simulink model "spring_mass_model_01"  (R2014a)
settings: Solver=FixedStepDiscrete  StartTime=0.0  StopTime=inf  FixedStep=sample_time  RelTol=1e-3
values from neighbouring files (symbols this model uses):
  sample_time = 1/update_freq    (= 0.001)    [init_spring_mass_model_01.m]
undefined symbols (not defined in the file or in its folder): boom_mount_angle, c_energy, contact_threshold, control_start_time, d_y_boom_com_offset, d_y_boom_hip_offset, d_y_mount_to_com, desired_torso_angle, DiscIntNeverNeededParam, dt_thrust, dx_avg_desired, extra_leg_damping, F_thrust, fcut_contact, ff_energy_l, ff_energy_r, g, g_reduced, h_boom, i_limit_lateral, initial_com_height, initial_dt, initial_dx, j_leg, k0_virtual, k_placement, k_sea, kd_flight, kd_lateral, kd_leg_angle, kd_leg_length_secondary, kd_torso, kd_virtual, ki_lateral, kp_flight_max, kp_flight_min, kp_lateral, kp_leg_angle, kp_leg_length_secondary, kp_torso, kp_virtual, l0_virtual, l_boom, l_boom_projected, l_max, l_min, l_retract, l_seg, lambda1, lambda2, lateral_offset, LEG_MTR_MAX_TORQUE, loaded_threshold, m_leg_motor, m_total_real, max_k_virtual, max_leg_angle, max_torque_lateral, min_k_virtual, min_leg_angle ... (+6)
libraries: simulink x22
(part 2 of 2)

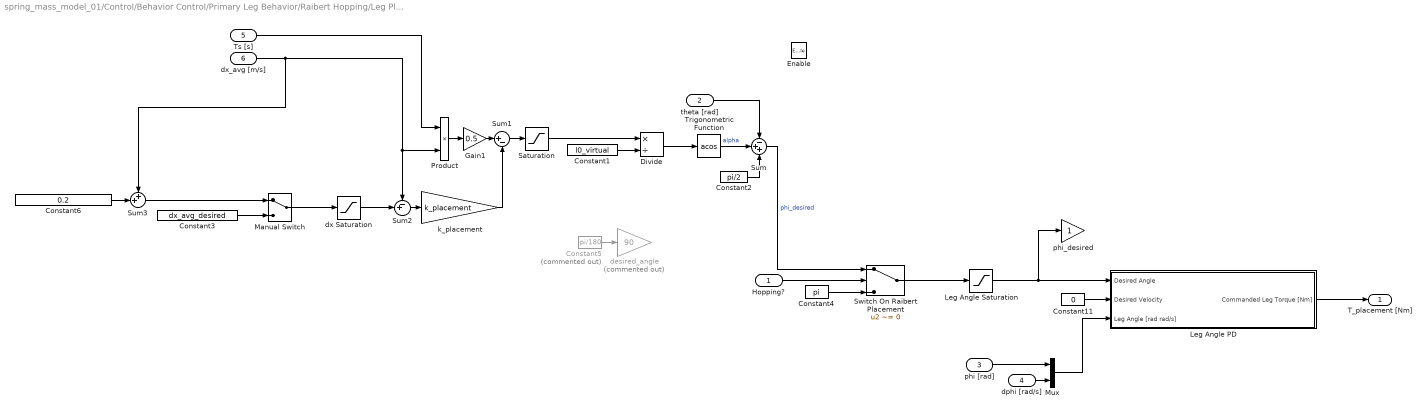
== system spring_mass_model_01/Control/Behavior Control/Primary Leg Behavior/Raibert Hopping/Leg Placement Torque ==
  Hopping? : Inport
  theta [rad] : Inport  Port=2
  phi [rad] : Inport  Port=3
  dphi [rad/s] : Inport  Port=4
  Ts [s] : Inport  Port=5
  dx_avg [m/s] : Inport  Port=6
  Enable : EnablePort  StatesWhenEnabling=reset
  Constant1 : Constant  Value=l0_virtual
  Constant11 : Constant  Value=0
  Constant2 : Constant  Value=pi/2
  Constant3 : Constant  Value=dx_avg_desired
  Constant4 : Constant  Value=pi
  Constant5 : Constant  Commented=on  Value=pi/180
  Constant6 : Constant  Value=0.2
  Divide : Product  Inputs=*/
  Gain1 : Gain  Gain=0.5
  Leg Angle PD : Subsystem
  Leg Angle Saturation : Saturate  UpperLimit=max_leg_angle  LowerLimit=min_leg_angle
      settings: AttributesFormatString=Hi: %<UpperLimit>\nLo: %<LowerLimit>
  Manual Switch : ManualSwitch
  Mux : Mux  Inputs=2
  Product : Product
  Saturation : Saturate  UpperLimit=x_limit  LowerLimit=-x_limit
      settings: AttributesFormatString=Hi: %<UpperLimit>\nLo: %<LowerLimit>
  Sum : Sum  Inputs=-++
  Sum1 : Sum  Inputs=|+-
  Sum2 : Sum  Inputs=-+|
  Sum3 : Sum  Inputs=++|
  Switch On Raibert Placement : Switch  Criteria=u2 ~= 0
  Trigonometric Function : Trigonometry  Operator=acos
  desired_angle : Gain  Commented=on  Gain=90
  dx Saturation : Saturate  UpperLimit=dx_avg_desired  LowerLimit=0
      settings: AttributesFormatString=Hi: %<UpperLimit>\nLo: %<LowerLimit>
  k_placement : Gain  Gain=k_placement
  phi_desired : Gain
  T_placement [Nm] : Outport  OutputWhenDisabled=reset  InitialOutput=[0]
  wires:
  Sum3/1 -> Manual Switch/1
  Constant6/1 -> Sum3/2
  dx_avg [m/s]/1 -> Product/2, Sum2/1, Sum3/1
  Constant3/1 -> Manual Switch/2
  Manual Switch/1 -> dx Saturation/1
  Switch On Raibert Placement/1 -> Leg Angle Saturation/1
  Constant5/1 -> desired_angle/1
  Leg Angle Saturation/1 -> Leg Angle PD/1(Desired Angle), phi_desired/1
  Hopping?/1 -> Switch On Raibert Placement/2
  Constant4/1 -> Switch On Raibert Placement/3
  dx Saturation/1 -> Sum2/2
  Sum2/1 -> k_placement/1
  k_placement/1 -> Sum1/2
  Sum1/1 -> Saturation/1
  Sum/1 -> Switch On Raibert Placement/1  "phi_desired"
  theta [rad]/1 -> Sum/1
  Constant2/1 -> Sum/3
  Trigonometric Function/1 -> Sum/2  "alpha"
  Divide/1 -> Trigonometric Function/1
  Constant1/1 -> Divide/2
  Saturation/1 -> Divide/1
  Gain1/1 -> Sum1/1
  Product/1 -> Gain1/1
  Ts [s]/1 -> Product/1
  dphi [rad/s]/1 -> Mux/2
  phi [rad]/1 -> Mux/1
  Leg Angle PD/1(Commanded Leg Torque [Nm]) -> T_placement [Nm]/1
  Mux/1 -> Leg Angle PD/3(Leg Angle [rad rad/s])
  Constant11/1 -> Leg Angle PD/2(Desired Velocity)

== system spring_mass_model_01/Control/Behavior Control/Primary Leg Behavior/Raibert Hopping/Leg Thrust ==
  Enable : EnablePort  StatesWhenEnabling=reset  ShowOutputPort=on
  F_thrust : Gain  Gain=F_thrust
  Thrust Timer : Subsystem
  thrust period? : simulink/Logic and Bit Operations/Compare To Constant  relop=<=  const=dt_thrust  OutDataTypeStr=uint8
  Thrust [N] : Outport  OutputWhenDisabled=reset  InitialOutput=[0]
  wires:
  thrust period?/1 -> F_thrust/1
  Enable/1 -> Thrust Timer/Enable
  Thrust Timer/1(timer [s]) -> thrust period?/1
  F_thrust/1 -> Thrust [N]/1

== system spring_mass_model_01/Control/Behavior Control/Primary Leg Behavior/Raibert Hopping/Nonlinear Spring Stiffness ==
  Right/Left [1/0] : Inport
  dl_virtual [m/s] : Inport  Port=2
  E_target1 : Constant  Value=ff_energy_r
  E_target2 : Constant  Value=ff_energy_l
  Product : Product  Inputs=3
  Saturation : Saturate  UpperLimit=max_k_virtual  LowerLimit=min_k_virtual  ZeroCross=off
  Sum : Sum  Inputs=+|-
  Sum2 : Sum  Inputs=--|
  Switch1 : Switch  Criteria=u2 ~= 0
  c_energy : Constant  Value=c_energy
  c_energy1 : Constant  Value=raibert_energy_injection
  k0_virtual : Constant  Value=k0_virtual
  k_virtual [N/m] : Outport
  wires:
  Product/1 -> Sum/2
  Sum/1 -> Saturation/1
  Saturation/1 -> k_virtual [N/m]/1
  k0_virtual/1 -> Sum/1
  c_energy/1 -> Product/3
  dl_virtual [m/s]/1 -> Product/2
  E_target1/1 -> Switch1/1
  E_target2/1 -> Switch1/3
  Right/Left [1/0]/1 -> Switch1/2
  Switch1/1 -> Sum2/2
  c_energy1/1 -> Sum2/1
  Sum2/1 -> Product/1

== system spring_mass_model_01/Control/Behavior Control/Primary Leg Behavior/Raibert Hopping/Trunk Balance PD Compensation ==
  Torso Pitch [rad rad/s] : Inport
  Enable : EnablePort  StatesWhenEnabling=reset
  Constant2 : Constant  Value=0
  Demux : Demux  Outputs=2
  Derivative Gain : Gain  Gain=kd_torso
  Gain1 : Gain  Gain=-1
  Proportional Gain : Gain  Gain=kp_torso
  Reference Lean [rad] : Constant  Value=desired_torso_angle
  Sum1 : Sum  Inputs=|+-
  Sum4 : Sum  Inputs=|+-
  Sum5 : Sum
  Torque [Nm] : Outport  OutputWhenDisabled=reset  InitialOutput=[0]
  wires:
  Gain1/1 -> Torque [Nm]/1
  Sum1/1 -> Derivative Gain/1
  Proportional Gain/1 -> Sum5/1
  Derivative Gain/1 -> Sum5/2
  Torso Pitch [rad rad/s]/1 -> Demux/1
  Sum4/1 -> Proportional Gain/1
  Demux/1 -> Sum4/2
  Reference Lean [rad]/1 -> Sum4/1
  Constant2/1 -> Sum1/1
  Demux/2 -> Sum1/2
  Sum5/1 -> Gain1/1

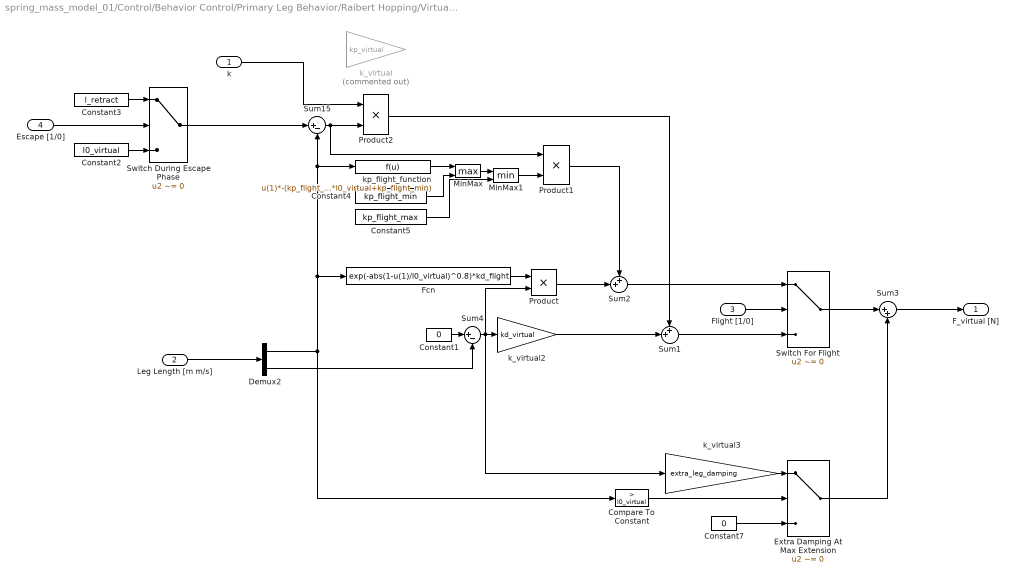
== system spring_mass_model_01/Control/Behavior Control/Primary Leg Behavior/Raibert Hopping/Virtual Leg Force and Swing Leg Retraction ==
  k : Inport
  Leg Length [m m/s] : Inport  Port=2
  Flight [1/0] : Inport  Port=3
  Escape [1/0] : Inport  Port=4
  Compare To Constant : simulink/Logic and Bit Operations/Compare To Constant  relop=>  const=l0_virtual  OutDataTypeStr=boolean
  Constant1 : Constant  Value=0
  Constant2 : Constant  Value=l0_virtual
  Constant3 : Constant  Value=l_retract
  Constant4 : Constant  Value=kp_flight_min
  Constant5 : Constant  Value=kp_flight_max
  Constant7 : Constant  Value=0
  Demux2 : Demux  Outputs=2
  Extra Damping At Max Extension : Switch  Criteria=u2 ~= 0
  Fcn : Fcn  Expr=exp(-abs(1-u(1)/l0_virtual)^0.8)*kd_flight
  MinMax : MinMax  Function=max  Inputs=2
  MinMax1 : MinMax  Inputs=2
  Product : Product
  Product1 : Product
  Product2 : Product
  Sum1 : Sum  Inputs=++|
  Sum15 : Sum  Inputs=|+-
  Sum2 : Sum  Inputs=++|
  Sum3 : Sum  Inputs=|++
  Sum4 : Sum  Inputs=|+-
  Switch During Escape Phase : Switch  Criteria=u2 ~= 0
  Switch For Flight : Switch  Criteria=u2 ~= 0
  k_virtual : Gain  Commented=on  Gain=kp_virtual
  k_virtual2 : Gain  Gain=kd_virtual
  k_virtual3 : Gain  Gain=extra_leg_damping
  kp_flight_function : Fcn  Expr=u(1)*-(kp_flight_max - kp_flight_min)/(l0_virtual - l_min)+((kp_flight_max - kp_flight_min)/(l0_virtual - l_min)*l0_virtual+kp_flight_min)
  F_virtual [N] : Outport
  wires:
  k_virtual3/1 -> Extra Damping At Max Extension/1
  Sum3/1 -> F_virtual [N]/1
  Extra Damping At Max Extension/1 -> Sum3/2
  Constant7/1 -> Extra Damping At Max Extension/3
  Compare To Constant/1 -> Extra Damping At Max Extension/2
  Switch During Escape Phase/1 -> Sum15/1
  Constant5/1 -> MinMax1/2
  MinMax1/1 -> Product1/2
  Constant4/1 -> MinMax/2
  MinMax/1 -> MinMax1/1
  Product1/1 -> Sum2/1
  kp_flight_function/1 -> MinMax/1
  Fcn/1 -> Product/1
  Sum15/1 -> Product2/2, Product1/1
  Leg Length [m m/s]/1 -> Demux2/1
  Demux2/1 -> Compare To Constant/1, Fcn/1, Sum15/2, kp_flight_function/1
  Sum1/1 -> Switch For Flight/3
  Constant1/1 -> Sum4/1
  Demux2/2 -> Sum4/2
  Product2/1 -> Sum1/1
  Sum4/1 -> k_virtual2/1, Product/2, k_virtual3/1
  k_virtual2/1 -> Sum1/2
  Flight [1/0]/1 -> Switch For Flight/2
  Escape [1/0]/1 -> Switch During Escape Phase/2
  Constant2/1 -> Switch During Escape Phase/3
  Constant3/1 -> Switch During Escape Phase/1
  Product/1 -> Sum2/2
  Switch For Flight/1 -> Sum3/1
  Sum2/1 -> Switch For Flight/1
  k/1 -> Product2/1

== system spring_mass_model_01/Control/Behavior Control/Primary Leg Behavior/SMM 01/COM Spring Angle Target Control 30kg Counterweight k=23000 1.5 m//s, 1.1204 target height 445.6 joules ==
  note: Angle of Attack Control Law From Poincare Map Method
  tFall [s] : Inport
  AlphaRef0 : Constant  Value=1.1989
  AlphaRef1 : Constant  Value=5*pi/4
  Compare To Constant : simulink/Logic and Bit Operations/Compare To Constant  relop=>  const=0  OutDataTypeStr=boolean  ZeroCross=off
  Compare To Constant1 : simulink/Logic and Bit Operations/Compare To Constant  relop=<  const=0.758998  OutDataTypeStr=boolean  ZeroCross=off
  Demux : Demux  Outputs=3
  Mux : Mux  Inputs=3
  Sum : Sum  Inputs=++|
  Switch : Switch  Criteria=u2 ~= 0
  Varying Component : Subsystem
  AlphaRef(t) [rad] : Outport
  dAlphaRef(t) [rad/s] : Outport  Port=2
  ddAlphaRef(t) [rad/s^2] : Outport  Port=3
  wires:
  tFall [s]/1 -> Compare To Constant/1, Compare To Constant1/1, Varying Component/1(tFall)
  Varying Component/2(dAlphaRef(t)) -> Mux/2
  Varying Component/3(ddAlphaRef(t)) -> Mux/3
  Compare To Constant/1 -> Varying Component/Enable
  Varying Component/1(AlphaRef(t)) -> Sum/2
  Sum/1 -> Mux/1
  AlphaRef0/1 -> Sum/1
  Compare To Constant1/1 -> Switch/2
  Mux/1 -> Switch/1
  Switch/1 -> Demux/1
  Demux/1 -> AlphaRef(t) [rad]/1
  Demux/2 -> dAlphaRef(t) [rad/s]/1
  Demux/3 -> ddAlphaRef(t) [rad/s^2]/1
  AlphaRef1/1 -> Switch/3

== system spring_mass_model_01/Control/Behavior Control/Primary Leg Behavior/SMM 01/COM Spring Angle Target Control 30kg Counterweight k=23000 l0=0.93 1.0 m//s, 0.99m target height 347.7454 joules ==
  note: Angle of Attack Control Law From Poincare Map Method
  tFall [s] : Inport
  AlphaRef0 : Constant  Value=1.0916
  AlphaRef1 : Constant  Value=3*pi/4
  Compare To Constant : simulink/Logic and Bit Operations/Compare To Constant  relop=>  const=0  OutDataTypeStr=boolean  ZeroCross=off
  Compare To Constant1 : simulink/Logic and Bit Operations/Compare To Constant  relop=<  const=0.423081  OutDataTypeStr=boolean  ZeroCross=off
  Demux : Demux  Outputs=3
  Mux : Mux  Inputs=3
  Sum : Sum  Inputs=++|
  Switch : Switch  Criteria=u2 ~= 0
  Varying Component : Subsystem
  AlphaRef(t) [rad] : Outport
  dAlphaRef(t) [rad/s] : Outport  Port=2
  ddAlphaRef(t) [rad/s^2] : Outport  Port=3
  wires:
  tFall [s]/1 -> Compare To Constant/1, Compare To Constant1/1, Varying Component/1(tFall)
  Varying Component/2(dAlphaRef(t)) -> Mux/2
  Varying Component/3(ddAlphaRef(t)) -> Mux/3
  Compare To Constant/1 -> Varying Component/Enable
  Varying Component/1(AlphaRef(t)) -> Sum/2
  Sum/1 -> Mux/1
  AlphaRef0/1 -> Sum/1
  Compare To Constant1/1 -> Switch/2
  Mux/1 -> Switch/1
  Switch/1 -> Demux/1
  Demux/1 -> AlphaRef(t) [rad]/1
  Demux/2 -> dAlphaRef(t) [rad/s]/1
  Demux/3 -> ddAlphaRef(t) [rad/s^2]/1
  AlphaRef1/1 -> Switch/3

== system spring_mass_model_01/Control/Behavior Control/Primary Leg Behavior/SMM 01/COM Spring Angle Target Control 30kg Counterweight k=23000 l0=0.95 0.3 m//s, 1.03m target height 332.0481 joules ==
  note: Angle of Attack Control Law From Poincare Map Method
  tFall [s] : Inport
  AlphaRef0 : Constant  Value=0.87325
  AlphaRef1 : Constant  Value=152*pi/180
  Compare To Constant : simulink/Logic and Bit Operations/Compare To Constant  relop=>  const=0  OutDataTypeStr=boolean  ZeroCross=off
  Compare To Constant1 : simulink/Logic and Bit Operations/Compare To Constant  relop=<  const=0.29581997557  OutDataTypeStr=boolean  ZeroCross=off
  Demux : Demux  Outputs=3
  Mux : Mux  Inputs=3
  Sum : Sum  Inputs=++|
  Switch : Switch  Criteria=u2 ~= 0
  Varying Component : Subsystem
  AlphaRef(t) [rad] : Outport
  dAlphaRef(t) [rad/s] : Outport  Port=2
  ddAlphaRef(t) [rad/s^2] : Outport  Port=3
  wires:
  tFall [s]/1 -> Compare To Constant/1, Compare To Constant1/1, Varying Component/1(tFall)
  Varying Component/2(dAlphaRef(t)) -> Mux/2
  Varying Component/3(ddAlphaRef(t)) -> Mux/3
  Compare To Constant/1 -> Varying Component/Enable
  Varying Component/1(AlphaRef(t)) -> Sum/2
  Sum/1 -> Mux/1
  AlphaRef0/1 -> Sum/1
  Compare To Constant1/1 -> Switch/2
  Mux/1 -> Switch/1
  Switch/1 -> Demux/1
  Demux/1 -> AlphaRef(t) [rad]/1
  Demux/2 -> dAlphaRef(t) [rad/s]/1
  Demux/3 -> ddAlphaRef(t) [rad/s^2]/1
  AlphaRef1/1 -> Switch/3

== system spring_mass_model_01/Control/Behavior Control/Primary Leg Behavior/SMM 01/COM Spring Angle Target Control 30kg Counterweight k=23000 l0=0.95 0.5 m//s, 1.03m target height 337.0561 joules ==
  note: Angle of Attack Control Law From Poincare Map Method
  tFall [s] : Inport
  AlphaRef0 : Constant  Value=0.91853
  AlphaRef1 : Constant  Value=3*pi/4
  Compare To Constant : simulink/Logic and Bit Operations/Compare To Constant  relop=>  const=0  OutDataTypeStr=boolean  ZeroCross=off
  Compare To Constant1 : simulink/Logic and Bit Operations/Compare To Constant  relop=<  const=0.309081155  OutDataTypeStr=boolean  ZeroCross=off
  Demux : Demux  Outputs=3
  Mux : Mux  Inputs=3
  Sum : Sum  Inputs=++|
  Switch : Switch  Criteria=u2 ~= 0
  Varying Component : Subsystem
  AlphaRef(t) [rad] : Outport
  dAlphaRef(t) [rad/s] : Outport  Port=2
  ddAlphaRef(t) [rad/s^2] : Outport  Port=3
  wires:
  tFall [s]/1 -> Compare To Constant/1, Compare To Constant1/1, Varying Component/1(tFall)
  Varying Component/2(dAlphaRef(t)) -> Mux/2
  Varying Component/3(ddAlphaRef(t)) -> Mux/3
  Compare To Constant/1 -> Varying Component/Enable
  Varying Component/1(AlphaRef(t)) -> Sum/2
  Sum/1 -> Mux/1
  AlphaRef0/1 -> Sum/1
  Compare To Constant1/1 -> Switch/2
  Mux/1 -> Switch/1
  Switch/1 -> Demux/1
  Demux/1 -> AlphaRef(t) [rad]/1
  Demux/2 -> dAlphaRef(t) [rad/s]/1
  Demux/3 -> ddAlphaRef(t) [rad/s^2]/1
  AlphaRef1/1 -> Switch/3

== system spring_mass_model_01/Control/Behavior Control/Primary Leg Behavior/SMM 01/COM Spring Angle Target Control 30kg Counterweight k=23000 l0=0.95 0.5 m//s, 1m target height 327.4669 joules ==
  note: Angle of Attack Control Law From Poincare Map Method
  tFall [s] : Inport
  AlphaRef0 : Constant  Value=0.95912
  AlphaRef1 : Constant  Value=1.883
  Compare To Constant : simulink/Logic and Bit Operations/Compare To Constant  relop=>  const=0  OutDataTypeStr=boolean  ZeroCross=off
  Compare To Constant1 : simulink/Logic and Bit Operations/Compare To Constant  relop=<  const=0.266  OutDataTypeStr=boolean  ZeroCross=off
  Demux : Demux  Outputs=3
  Mux : Mux  Inputs=3
  Sum : Sum  Inputs=++|
  Switch : Switch  Criteria=u2 ~= 0
  Varying Component : Subsystem
  AlphaRef(t) [rad] : Outport
  dAlphaRef(t) [rad/s] : Outport  Port=2
  ddAlphaRef(t) [rad/s^2] : Outport  Port=3
  wires:
  AlphaRef1/1 -> Switch/3
  Demux/3 -> ddAlphaRef(t) [rad/s^2]/1
  Demux/2 -> dAlphaRef(t) [rad/s]/1
  Demux/1 -> AlphaRef(t) [rad]/1
  Switch/1 -> Demux/1
  Mux/1 -> Switch/1
  Compare To Constant1/1 -> Switch/2
  AlphaRef0/1 -> Sum/1
  Sum/1 -> Mux/1
  Varying Component/1(AlphaRef(t)) -> Sum/2
  Compare To Constant/1 -> Varying Component/Enable
  Varying Component/3(ddAlphaRef(t)) -> Mux/3
  Varying Component/2(dAlphaRef(t)) -> Mux/2
  tFall [s]/1 -> Varying Component/1(tFall), Compare To Constant1/1, Compare To Constant/1

== system spring_mass_model_01/Control/Behavior Control/Primary Leg Behavior/SMM 01/COM Spring Angle Target Control 30kg Counterweight k=23000 l0=0.95 1.0 m//s, 1.03m target height 360.5311 joules ==
  note: Angle of Attack Control Law From Poincare Map Method
  tFall [s] : Inport
  AlphaRef0 : Constant  Value=1.0551
  AlphaRef1 : Constant  Value=3*pi/4
  Compare To Constant : simulink/Logic and Bit Operations/Compare To Constant  relop=>  const=0  OutDataTypeStr=boolean  ZeroCross=off
  Compare To Constant1 : simulink/Logic and Bit Operations/Compare To Constant  relop=<  const=0.43285  OutDataTypeStr=boolean  ZeroCross=off
  Demux : Demux  Outputs=3
  Mux : Mux  Inputs=3
  Sum : Sum  Inputs=++|
  Switch : Switch  Criteria=u2 ~= 0
  Varying Component : Subsystem
  AlphaRef(t) [rad] : Outport
  dAlphaRef(t) [rad/s] : Outport  Port=2
  ddAlphaRef(t) [rad/s^2] : Outport  Port=3
  wires:
  AlphaRef1/1 -> Switch/3
  Demux/3 -> ddAlphaRef(t) [rad/s^2]/1
  Demux/2 -> dAlphaRef(t) [rad/s]/1
  Demux/1 -> AlphaRef(t) [rad]/1
  Switch/1 -> Demux/1
  Mux/1 -> Switch/1
  Compare To Constant1/1 -> Switch/2
  AlphaRef0/1 -> Sum/1
  Sum/1 -> Mux/1
  Varying Component/1(AlphaRef(t)) -> Sum/2
  Compare To Constant/1 -> Varying Component/Enable
  Varying Component/3(ddAlphaRef(t)) -> Mux/3
  Varying Component/2(dAlphaRef(t)) -> Mux/2
  tFall [s]/1 -> Varying Component/1(tFall), Compare To Constant1/1, Compare To Constant/1

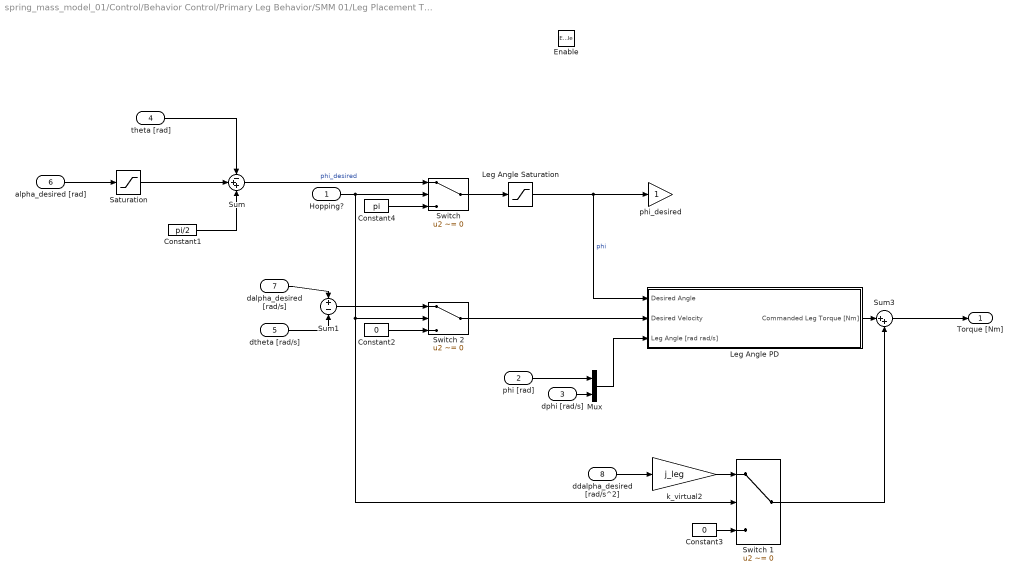
== system spring_mass_model_01/Control/Behavior Control/Primary Leg Behavior/SMM 01/Leg Placement Torque ==
  Hopping? : Inport
  phi [rad] : Inport  Port=2
  dphi [rad/s] : Inport  Port=3
  theta [rad] : Inport  Port=4
  dtheta [rad/s] : Inport  Port=5
  alpha_desired [rad] : Inport  Port=6
  dalpha_desired [rad/s] : Inport  Port=7
  ddalpha_desired [rad/s^2] : Inport  Port=8
  Enable : EnablePort  StatesWhenEnabling=reset
  Constant1 : Constant  Value=pi/2
  Constant2 : Constant  Value=0
  Constant3 : Constant  Value=0
  Constant4 : Constant  Value=pi
  Leg Angle PD : Subsystem
  Leg Angle Saturation : Saturate  UpperLimit=max_leg_angle  LowerLimit=min_leg_angle
      settings: AttributesFormatString=Hi: %<UpperLimit>\nLo: %<LowerLimit>
  Mux : Mux  Inputs=2
  Saturation : Saturate  UpperLimit=110*pi/180  LowerLimit=70*pi/180
      settings: AttributesFormatString=|
      | Hi: %<UpperLimit>
      | Lo: %<LowerLimit>
  Sum : Sum  Inputs=-++
  Sum1 : Sum  Inputs=+|-
  Sum3 : Sum  Inputs=|++
  Switch : Switch  Criteria=u2 ~= 0
  Switch 1 : Switch  Criteria=u2 ~= 0
  Switch 2 : Switch  Criteria=u2 ~= 0
  k_virtual2 : Gain  Gain=j_leg
  phi_desired : Gain
  Torque [Nm] : Outport  OutputWhenDisabled=reset  InitialOutput=[0]
  wires:
  Leg Angle Saturation/1 -> Leg Angle PD/1(Desired Angle), phi_desired/1  "phi"
  phi [rad]/1 -> Mux/1
  Mux/1 -> Leg Angle PD/3(Leg Angle [rad rad/s])
  Switch 2/1 -> Leg Angle PD/2(Desired Velocity)
  Sum3/1 -> Torque [Nm]/1
  ddalpha_desired [rad/s^2]/1 -> k_virtual2/1
  Leg Angle PD/1(Commanded Leg Torque [Nm]) -> Sum3/1
  dphi [rad/s]/1 -> Mux/2
  Sum/1 -> Switch/1  "phi_desired"
  Switch/1 -> Leg Angle Saturation/1
  Constant4/1 -> Switch/3
  Hopping?/1 -> Switch 1/2, Switch 2/2, Switch/2
  Constant1/1 -> Sum/3
  alpha_desired [rad]/1 -> Saturation/1
  theta [rad]/1 -> Sum/1
  dalpha_desired [rad/s]/1 -> Sum1/1
  dtheta [rad/s]/1 -> Sum1/2
  Constant2/1 -> Switch 2/3
  Sum1/1 -> Switch 2/1
  Constant3/1 -> Switch 1/3
  k_virtual2/1 -> Switch 1/1
  Switch 1/1 -> Sum3/2
  Saturation/1 -> Sum/2

== system spring_mass_model_01/Control/Behavior Control/Primary Leg Behavior/SMM 01/Nonlinear Spring Stiffness ==
  Energy Error [J] : Inport
  dl_virtual [m/s] : Inport  Port=2
  Product : Product  Inputs=3
  Saturation : Saturate  UpperLimit=max_k_virtual  LowerLimit=min_k_virtual  ZeroCross=off
  Sum : Sum  Inputs=+|-
  c_energy : Constant  Value=c_energy
  k0_virtual : Constant  Value=k0_virtual
  k_virtual [N/m] : Outport
  wires:
  Product/1 -> Sum/2
  Sum/1 -> Saturation/1
  Saturation/1 -> k_virtual [N/m]/1
  Energy Error [J]/1 -> Product/1
  k0_virtual/1 -> Sum/1
  c_energy/1 -> Product/3
  dl_virtual [m/s]/1 -> Product/2

== system spring_mass_model_01/Control/Behavior Control/Primary Leg Behavior/SMM 01/Trunk Balance PD Compensation ==
  Torso Pitch [rad rad/s] : Inport
  Enable : EnablePort  StatesWhenEnabling=reset
  Constant2 : Constant  Value=0
  Demux : Demux  Outputs=2
  Derivative Gain : Gain  Gain=kd_torso
  Gain1 : Gain  Gain=-1
  Proportional Gain : Gain  Gain=kp_torso
  Reference Lean [rad] : Constant  Value=desired_torso_angle
  Sum1 : Sum  Inputs=|+-
  Sum4 : Sum  Inputs=|+-
  Sum5 : Sum
  Torque [Nm] : Outport  OutputWhenDisabled=reset  InitialOutput=[0]
  wires:
  Gain1/1 -> Torque [Nm]/1
  Sum1/1 -> Derivative Gain/1
  Proportional Gain/1 -> Sum5/1
  Derivative Gain/1 -> Sum5/2
  Torso Pitch [rad rad/s]/1 -> Demux/1
  Sum4/1 -> Proportional Gain/1
  Demux/1 -> Sum4/2
  Reference Lean [rad]/1 -> Sum4/1
  Constant2/1 -> Sum1/1
  Demux/2 -> Sum1/2
  Sum5/1 -> Gain1/1

== system spring_mass_model_01/Control/Behavior Control/Primary Leg Behavior/SMM 01/Virtual Leg Force and Swing Leg Retraction ==
  k_virtual [N/m] : Inport
  Leg Length [m m/s] : Inport  Port=2
  Flight [1/0] : Inport  Port=3
  Escape [1/0] : Inport  Port=4
  Demux1 : Demux  Outputs=2
  Hold Initial : Subsystem
  Logical Operator : Logic  Operator=NOT  IconShape=distinctive  AllPortsSameDT=off  OutDataTypeStr=boolean
  Virtual Spring Force : MATLAB Function  TreatAsAtomicUnit=on
  F_virtual [N] : Outport
  wires:
  Virtual Spring Force/1(F_virtual) -> F_virtual [N]/1
  Logical Operator/1 -> Hold Initial/Trigger
  Hold Initial/1(out) -> Virtual Spring Force/4(l_virtual_initial)
  Flight [1/0]/1 -> Virtual Spring Force/1(flight), Logical Operator/1
  Demux1/1 -> Hold Initial/1(in), Virtual Spring Force/5(l_spring)
  Leg Length [m m/s]/1 -> Demux1/1
  Demux1/2 -> Virtual Spring Force/6(dl_spring)
  Escape [1/0]/1 -> Virtual Spring Force/2(escape)
  k_virtual [N/m]/1 -> Virtual Spring Force/3(k_virtual)

== system spring_mass_model_01/Control/Behavior Control/Primary Leg Behavior/Raibert Hopping/Leg Placement Torque/Leg Angle PD ==
  Desired Angle : Inport
  Desired Velocity : Inport  Port=2
  Leg Angle [rad rad/s] : Inport  Port=3
  Demux1 : Demux  Outputs=2
  Sum7 : Sum  Inputs=|+-
  Sum8 : Sum  Inputs=|+-
  Sum9 : Sum
  kd_leg_angle : Gain  Gain=kd_leg_angle
  kp_leg_angle : Gain  Gain=kp_leg_angle
  Commanded Leg Torque [Nm] : Outport
  wires:
  kp_leg_angle/1 -> Sum9/1
  Sum7/1 -> kp_leg_angle/1
  Demux1/1 -> Sum7/2
  Sum9/1 -> Commanded Leg Torque [Nm]/1
  Desired Velocity/1 -> Sum8/1
  Sum8/1 -> kd_leg_angle/1
  Desired Angle/1 -> Sum7/1
  kd_leg_angle/1 -> Sum9/2
  Demux1/2 -> Sum8/2
  Leg Angle [rad rad/s]/1 -> Demux1/1

== system spring_mass_model_01/Control/Behavior Control/Primary Leg Behavior/Raibert Hopping/Leg Thrust/Thrust Timer ==
  Enable : EnablePort  StatesWhenEnabling=reset  ShowOutputPort=on
  Constant : Constant
  Discrete-Time Integrator : DiscreteIntegrator  IntegratorMethod=Accumulation: Forward Euler  gainval=sample_time  ExternalReset=rising  SampleTime=sample_time  ICPrevOutput=DiscIntNeverNeededParam  ICPrevScaledInput=DiscIntNeverNeededParam
  timer [s] : Outport  InitialOutput=[0]
  wires:
  Constant/1 -> Discrete-Time Integrator/1
  Enable/1 -> Discrete-Time Integrator/2
  Discrete-Time Integrator/1 -> timer [s]/1

== system spring_mass_model_01/Control/Behavior Control/Primary Leg Behavior/SMM 01/COM Spring Angle Target Control 30kg Counterweight k=23000 1.5 m//s, 1.1204 target height 445.6 joules/Varying Component ==
  tFall : Inport
  Enable : EnablePort  StatesWhenEnabling=reset  ZeroCross=off
      settings: AttributesFormatString=When enabled: %<StatesWhenEnabling>
  AlphaRef(t) Control Law for 1m : Fcn  Expr=6.1973*u^3-2.4174*u^2+1.859*u
  acceleration of AlphaRef(t) Control Law for 1m : Fcn  Expr=2*3*6.1973*u-2*2.4174
  velocity of AlphaRef(t) Control Law for 1m : Fcn  Expr=3*6.1973*u^2-2*2.4174*u+1.859
  AlphaRef(t) : Outport  OutputWhenDisabled=reset  InitialOutput=0
      settings: AttributesFormatString=When disabled: %<OutputWhenDisabled>\nDisabled Output: %<InitialOutput>
  dAlphaRef(t) : Outport  Port=2  OutputWhenDisabled=reset  InitialOutput=0
      settings: AttributesFormatString=When disbaled: %<OutputWhenDisabled>\nDisabled output: %<InitialOutput>
  ddAlphaRef(t) : Outport  Port=3  OutputWhenDisabled=reset  InitialOutput=0
      settings: AttributesFormatString=When disabled: %<OutputWhenDisabled>\nDisabled output: %<InitialOutput>
  wires:
  tFall/1 -> AlphaRef(t) Control Law for 1m/1, velocity of AlphaRef(t) Control Law for 1m/1, acceleration of AlphaRef(t) Control Law for 1m/1
  AlphaRef(t) Control Law for 1m/1 -> AlphaRef(t)/1
  velocity of AlphaRef(t) Control Law for 1m/1 -> dAlphaRef(t)/1
  acceleration of AlphaRef(t) Control Law for 1m/1 -> ddAlphaRef(t)/1

== system spring_mass_model_01/Control/Behavior Control/Primary Leg Behavior/SMM 01/COM Spring Angle Target Control 30kg Counterweight k=23000 l0=0.93 1.0 m//s, 0.99m target height 347.7454 joules/Varying Component ==
  tFall : Inport
  Enable : EnablePort  StatesWhenEnabling=reset  ZeroCross=off
      settings: AttributesFormatString=When enabled: %<StatesWhenEnabling>
  AlphaRef(t) Control Law for 1m : Fcn  Expr=9.278*u^3 -3.1458*u^2+2.6592*u
  acceleration of AlphaRef(t) Control Law for 1m : Fcn  Expr=2*3*9.278*u -2*3.1458
  velocity of AlphaRef(t) Control Law for 1m : Fcn  Expr=3*9.278*u^2 -2*3.1458*u+2.6592
  AlphaRef(t) : Outport  OutputWhenDisabled=reset  InitialOutput=0
      settings: AttributesFormatString=When disabled: %<OutputWhenDisabled>\nDisabled Output: %<InitialOutput>
  dAlphaRef(t) : Outport  Port=2  OutputWhenDisabled=reset  InitialOutput=0
      settings: AttributesFormatString=When disbaled: %<OutputWhenDisabled>\nDisabled output: %<InitialOutput>
  ddAlphaRef(t) : Outport  Port=3  OutputWhenDisabled=reset  InitialOutput=0
      settings: AttributesFormatString=When disabled: %<OutputWhenDisabled>\nDisabled output: %<InitialOutput>
  wires:
  tFall/1 -> AlphaRef(t) Control Law for 1m/1, velocity of AlphaRef(t) Control Law for 1m/1, acceleration of AlphaRef(t) Control Law for 1m/1
  AlphaRef(t) Control Law for 1m/1 -> AlphaRef(t)/1
  velocity of AlphaRef(t) Control Law for 1m/1 -> dAlphaRef(t)/1
  acceleration of AlphaRef(t) Control Law for 1m/1 -> ddAlphaRef(t)/1

== system spring_mass_model_01/Control/Behavior Control/Primary Leg Behavior/SMM 01/COM Spring Angle Target Control 30kg Counterweight k=23000 l0=0.95 0.3 m//s, 1.03m target height 332.0481 joules/Varying Component ==
  tFall : Inport
  Enable : EnablePort  StatesWhenEnabling=reset  ZeroCross=off
      settings: AttributesFormatString=When enabled: %<StatesWhenEnabling>
  AlphaRef(t) Control Law for 1m : Fcn  Expr=-3764.4*u^5 + 2183.9*u^4 - 375.78*u^3 + 34.379*u^2 + 1.023*u
  acceleration of AlphaRef(t) Control Law for 1m : Fcn  Expr=-4*5*3764.4*u^3 + 3*4*2183.9*u^2 - 2*3*375.78*u + 2*34.379
  velocity of AlphaRef(t) Control Law for 1m : Fcn  Expr=-5*3764.4*u^4 + 4*2183.9*u^3 - 3*375.78*u^2 + 2*34.379*u + 1.023
  AlphaRef(t) : Outport  OutputWhenDisabled=reset  InitialOutput=0
      settings: AttributesFormatString=When disabled: %<OutputWhenDisabled>\nDisabled Output: %<InitialOutput>
  dAlphaRef(t) : Outport  Port=2  OutputWhenDisabled=reset  InitialOutput=0
      settings: AttributesFormatString=When disbaled: %<OutputWhenDisabled>\nDisabled output: %<InitialOutput>
  ddAlphaRef(t) : Outport  Port=3  OutputWhenDisabled=reset  InitialOutput=0
      settings: AttributesFormatString=When disabled: %<OutputWhenDisabled>\nDisabled output: %<InitialOutput>
  wires:
  tFall/1 -> AlphaRef(t) Control Law for 1m/1, velocity of AlphaRef(t) Control Law for 1m/1, acceleration of AlphaRef(t) Control Law for 1m/1
  AlphaRef(t) Control Law for 1m/1 -> AlphaRef(t)/1
  velocity of AlphaRef(t) Control Law for 1m/1 -> dAlphaRef(t)/1
  acceleration of AlphaRef(t) Control Law for 1m/1 -> ddAlphaRef(t)/1

== system spring_mass_model_01/Control/Behavior Control/Primary Leg Behavior/SMM 01/COM Spring Angle Target Control 30kg Counterweight k=23000 l0=0.95 0.5 m//s, 1.03m target height 337.0561 joules/Varying Component ==
  tFall : Inport
  Enable : EnablePort  StatesWhenEnabling=reset  ZeroCross=off
      settings: AttributesFormatString=When enabled: %<StatesWhenEnabling>
  AlphaRef(t) Control Law for 1m : Fcn  Expr=11.603*u^3 + 4.0244*u^2 + 2.2991*u
  acceleration of AlphaRef(t) Control Law for 1m : Fcn  Expr=2*3*11.603*u + 2*4.0244
  velocity of AlphaRef(t) Control Law for 1m : Fcn  Expr=3*11.603*u^2 + 2*4.0244*u + 2.2991
  AlphaRef(t) : Outport  OutputWhenDisabled=reset  InitialOutput=0
      settings: AttributesFormatString=When disabled: %<OutputWhenDisabled>\nDisabled Output: %<InitialOutput>
  dAlphaRef(t) : Outport  Port=2  OutputWhenDisabled=reset  InitialOutput=0
      settings: AttributesFormatString=When disbaled: %<OutputWhenDisabled>\nDisabled output: %<InitialOutput>
  ddAlphaRef(t) : Outport  Port=3  OutputWhenDisabled=reset  InitialOutput=0
      settings: AttributesFormatString=When disabled: %<OutputWhenDisabled>\nDisabled output: %<InitialOutput>
  wires:
  tFall/1 -> AlphaRef(t) Control Law for 1m/1, velocity of AlphaRef(t) Control Law for 1m/1, acceleration of AlphaRef(t) Control Law for 1m/1
  AlphaRef(t) Control Law for 1m/1 -> AlphaRef(t)/1
  velocity of AlphaRef(t) Control Law for 1m/1 -> dAlphaRef(t)/1
  acceleration of AlphaRef(t) Control Law for 1m/1 -> ddAlphaRef(t)/1

== system spring_mass_model_01/Control/Behavior Control/Primary Leg Behavior/SMM 01/COM Spring Angle Target Control 30kg Counterweight k=23000 l0=0.95 0.5 m//s, 1m target height 327.4669 joules/Varying Component ==
  tFall : Inport
  Enable : EnablePort  StatesWhenEnabling=reset  ZeroCross=off
      settings: AttributesFormatString=When enabled: %<StatesWhenEnabling>
  AlphaRef(t) Control Law for 1m : Fcn  Expr=-66.193*u^3 + 23.067*u^2 + 2.0228*u
  acceleration of AlphaRef(t) Control Law for 1m : Fcn  Expr=-2*3*66.193*u^2 + 2*23.067
  velocity of AlphaRef(t) Control Law for 1m : Fcn  Expr=-3*66.193*u^2 + 2*23.067*u + 2.0228
  AlphaRef(t) : Outport  OutputWhenDisabled=reset  InitialOutput=0
      settings: AttributesFormatString=When disabled: %<OutputWhenDisabled>\nDisabled Output: %<InitialOutput>
  dAlphaRef(t) : Outport  Port=2  OutputWhenDisabled=reset  InitialOutput=0
      settings: AttributesFormatString=When disbaled: %<OutputWhenDisabled>\nDisabled output: %<InitialOutput>
  ddAlphaRef(t) : Outport  Port=3  OutputWhenDisabled=reset  InitialOutput=0
      settings: AttributesFormatString=When disabled: %<OutputWhenDisabled>\nDisabled output: %<InitialOutput>
  wires:
  acceleration of AlphaRef(t) Control Law for 1m/1 -> ddAlphaRef(t)/1
  velocity of AlphaRef(t) Control Law for 1m/1 -> dAlphaRef(t)/1
  AlphaRef(t) Control Law for 1m/1 -> AlphaRef(t)/1
  tFall/1 -> acceleration of AlphaRef(t) Control Law for 1m/1, velocity of AlphaRef(t) Control Law for 1m/1, AlphaRef(t) Control Law for 1m/1

== system spring_mass_model_01/Control/Behavior Control/Primary Leg Behavior/SMM 01/COM Spring Angle Target Control 30kg Counterweight k=23000 l0=0.95 1.0 m//s, 1.03m target height 360.5311 joules/Varying Component ==
  tFall : Inport
  Enable : EnablePort  StatesWhenEnabling=reset  ZeroCross=off
      settings: AttributesFormatString=When enabled: %<StatesWhenEnabling>
  AlphaRef(t) Control Law for 1m : Fcn  Expr=8.306*u^3 -2.3503*u^2+2.467*u
  acceleration of AlphaRef(t) Control Law for 1m : Fcn  Expr=2*3*8.306*u^3 -2*2.3503
  velocity of AlphaRef(t) Control Law for 1m : Fcn  Expr=3*8.306*u^3 -2*2.3503*u+2.467
  AlphaRef(t) : Outport  OutputWhenDisabled=reset  InitialOutput=0
      settings: AttributesFormatString=When disabled: %<OutputWhenDisabled>\nDisabled Output: %<InitialOutput>
  dAlphaRef(t) : Outport  Port=2  OutputWhenDisabled=reset  InitialOutput=0
      settings: AttributesFormatString=When disbaled: %<OutputWhenDisabled>\nDisabled output: %<InitialOutput>
  ddAlphaRef(t) : Outport  Port=3  OutputWhenDisabled=reset  InitialOutput=0
      settings: AttributesFormatString=When disabled: %<OutputWhenDisabled>\nDisabled output: %<InitialOutput>
  wires:
  acceleration of AlphaRef(t) Control Law for 1m/1 -> ddAlphaRef(t)/1
  velocity of AlphaRef(t) Control Law for 1m/1 -> dAlphaRef(t)/1
  AlphaRef(t) Control Law for 1m/1 -> AlphaRef(t)/1
  tFall/1 -> acceleration of AlphaRef(t) Control Law for 1m/1, velocity of AlphaRef(t) Control Law for 1m/1, AlphaRef(t) Control Law for 1m/1

== system spring_mass_model_01/Control/Behavior Control/Primary Leg Behavior/SMM 01/Leg Placement Torque/Leg Angle PD ==
  Desired Angle : Inport
  Desired Velocity : Inport  Port=2
  Leg Angle [rad rad/s] : Inport  Port=3
  Demux1 : Demux  Outputs=2
  Sum7 : Sum  Inputs=|+-
  Sum8 : Sum  Inputs=|+-
  Sum9 : Sum
  kd_leg_angle : Gain  Gain=kd_leg_angle
  kp_leg_angle : Gain  Gain=kp_leg_angle
  Commanded Leg Torque [Nm] : Outport
  wires:
  kp_leg_angle/1 -> Sum9/1
  Sum7/1 -> kp_leg_angle/1
  Demux1/1 -> Sum7/2
  Sum9/1 -> Commanded Leg Torque [Nm]/1
  Desired Velocity/1 -> Sum8/1
  Sum8/1 -> kd_leg_angle/1
  Desired Angle/1 -> Sum7/1
  kd_leg_angle/1 -> Sum9/2
  Demux1/2 -> Sum8/2
  Leg Angle [rad rad/s]/1 -> Demux1/1

== system spring_mass_model_01/Control/Behavior Control/Primary Leg Behavior/SMM 01/Virtual Leg Force and Swing Leg Retraction/Hold Initial ==
  in : Inport
  Trigger : TriggerPort  ShowOutputPort=on  PortDimensions=1
  Subsystem : Subsystem
  out : Outport  InitialOutput=[0]
  wires:
  in/1 -> Subsystem/1(in)
  Subsystem/1(out) -> out/1
  Trigger/1 -> Subsystem/Enable

== system spring_mass_model_01/Control/Behavior Control/Primary Leg Behavior/SMM 01/Virtual Leg Force and Swing Leg Retraction/Hold Initial/Subsystem ==
  in : Inport
  Enable : EnablePort
  out : Outport
  wires:
  in/1 -> out/1

== stateflow chart spring_mass_model_01/Control/Behavior Control/Primary Leg Behavior/Raibert  Hopper State Machine ==
  state Loading
    entry: placement = 0;
    entry: posture = 0;
    entry: thrust = 0;
    entry: flight = 0;
    entry: escape = 0;
  state Compression
    entry: placement = 0;
    entry: posture = 1;
    entry: thrust = 0;
    entry: flight = 0;
    entry: escape = 0;
  state Thrust
    entry: placement = 0;
    entry: posture = 1;
    entry: thrust = 1;
    entry: flight = 0;
    entry: escape = 0;
  state Unloading
    entry: placement = 0;
    entry: posture = 0;
    entry: thrust = 1;
    entry: flight = 0;
    entry: escape = 0;
  state Escape
    entry: placement = 0;
    entry: posture = 0;
    entry: thrust = 0;
    entry: flight = 1;
    entry: escape = 1;
  state Flight
    entry: placement = 1;
    entry: posture = 0;
    entry: thrust = 0;
    entry: flight = 1;
    entry: escape = 0;
  (junction 91) -> Loading
  Loading -> (junction 130) [order 2] : [Fy < contact_threshold]
  (junction 93) -> (junction 91)
  (junction 130) -> (junction 128)
  Loading -> Compression [order 1] : [Fy > loaded_threshold]
  (junction 115) -> Compression
  (junction 118) -> (junction 115)
  Compression -> Thrust : [dl >= 0 && dl_prev < 0]
  Thrust -> Unloading [order 1] : [Fy < loaded_threshold]
  Thrust -> (junction 102) [order 2] : [l > l_max]
  (junction 102) -> (junction 100)
  (junction 122) -> (junction 118)
  Unloading -> Escape [order 1] : [Fy < contact_threshold || l > l_max]
  Unloading -> (junction 122) [order 2] : [Fy > loaded_threshold]
  Escape -> Flight : after(t_flight,sec)
  (junction 100) -> Escape
  (default) -> Flight
  Flight -> (junction 93) : [Fy > contact_threshold]
  (junction 128) -> Flight
  data: flight output; escape output; thrust output; posture output; l input; dl input; dl_prev input; Fy input; t_flight parameter; placement output; l_max parameter; contact_threshold parameter; loaded_threshold parameter

== matlab function spring_mass_model_01/Control/Behavior Control/Primary Leg Behavior/SMM 01/Virtual Leg Force and Swing Leg Retraction/Virtual Spring Force ==
  data: flight input; escape input; k_virtual input; l_virtual_initial input; l_spring input; F_virtual output; dl_spring input; l0_virtual parameter; l_retract parameter; kd_flight parameter; kp_flight_min parameter; kp_flight_max parameter
function F_virtual  = fcn(flight, escape, k_virtual, l_virtual_initial, l_spring, dl_spring, ...
                          l0_virtual, l_retract,...
                          kd_flight, kp_flight_min, kp_flight_max)
                          
  if flight == 1
    %% Flight
    l_target = l0_virtual;
    if escape == 1
      l_target = l_retract;
    end
    delta_l = l_target - l_spring;
    delta_dl = 0 - dl_spring;
    kp_flight = l_spring*-(kp_flight_max - kp_flight_min)/(l0_virtual - l_min)+((kp_flight_max - kp_flight_min)/(l0_virtual - l_min)*l0_virtual+kp_flight_min);
    kp_flight = min(max(kp_flight, kp_flight_min), kp_flight_max);
    kd_flight = exp(-abs(1-l_spring/l0_virtual)^0.8)*kd_flight;
    if l_spring > l0_virtual
        kd_flight = kd_flight + extra_leg_damping;
    end
    F_virtual = kp_flight*delta_l + kd_flight*delta_dl;
    
  else  
    %% Stance
    delta_l = l_virtual_initial - l_spring;
    delta_dl = 0 - dl_spring;
    F_virtual = k_virtual*delta_l + kd_virtual*delta_dl;
  end



end

== matlab function spring_mass_model_01/Control/Behavior Control/Torque Distribution Right/Motor Torque Saturation Optimization ==
  data: x1s input; t1 output; x2s input; lambda1 parameter; lambda2 parameter; LEG_MTR_MAX_TORQUE parameter; t2 output
% Optimal leg motor torque distribution
function [t1, t2] = distribute_torque(x1s, x2s, lambda1, lambda2, LEG_MTR_MAX_TORQUE)

s = LEG_MTR_MAX_TORQUE;

% possible solutions
x1 = [                                                      x1s;
                                                            0;
                                                            s;
                                                            0;
                                                           -s;
  (lambda2*s + lambda1*x1s - lambda2*x2s)/(lambda1 + lambda2);
  (lambda1*x1s - lambda2*s + lambda2*x2s)/(lambda1 + lambda2);
  (lambda2*s + lambda1*x1s + lambda2*x2s)/(lambda1 + lambda2);
 -(lambda2*s - lambda1*x1s + lambda2*x2s)/(lambda1 + lambda2)];
 
x2 = [                                                      x2s;
                                                            s;
                                                            0;
                                                           -s;
                                                            0;
  (lambda1*s - lambda1*x1s + lambda2*x2s)/(lambda1 + lambda2);
  (lambda1*s + lambda1*x1s + lambda2*x2s)/(lambda1 + lambda2);
  (lambda1*x1s - lambda1*s + lambda2*x2s)/(lambda1 + lambda2);
 -(lambda1*s + lambda1*x1s - lambda2*x2s)/(lambda1 + lambda2)];

% test constraints
c1 = s - x1 - x2 >= 0;
c2 = s + x1 + x2 >= 0;
c3 = s - x1 + x2 >= 0;
c4 = s + x1 - x2 >= 0;
constraints = c1 & c2 & c3 & c4;

% objective function to maximize
f = -lambda1*(x1-x1s).^2-lambda2*(x2-x2s).^2;
satisfied = find(constraints);
[~,I] = max(f(satisfied));

t1 = x1(satisfied(I));
t2 = x2(satisfied(I));

== matlab function spring_mass_model_01/Control/Behavior Control/Velocity Estimation/dx_and_dy_from_yaw_and_roll ==
  data: qRoll input; dqRoll input; dx output; dqYaw input; dqPitch input; l_boom parameter; l_boom_projected parameter; h_boom parameter; boom_mount_angle parameter; d_y_boom_com_offset parameter; d_y_boom_hip_offset parameter; dy output; d_y_mount_to_com parameter; y_com output; y_hip output
function [dx, dy, y_com, y_hip] = fcn(qRoll, dqRoll, dqYaw, dqPitch, ...
                        l_boom, l_boom_projected, h_boom, boom_mount_angle, ...
                        d_y_boom_com_offset, d_y_boom_hip_offset, d_y_mount_to_com)
    % dx
    x_boom = l_boom * cos(qRoll);
    x_mount_to_center = d_y_mount_to_com * sin(qRoll-boom_mount_angle);
    dx = dqYaw * (x_boom + x_mount_to_center) - dqPitch * d_y_mount_to_com;
    
    % dy
    dy    = dqRoll * l_boom_projected * cos(qRoll)  +  d_y_boom_com_offset * dqRoll * sin(qRoll-boom_mount_angle);
    
    % y (COM and hip point)
    y_com = h_boom + l_boom_projected * sin(qRoll)  -  d_y_boom_com_offset * cos(qRoll-boom_mount_angle); 
    y_hip = h_boom + l_boom_projected * sin(qRoll)  -  d_y_boom_hip_offset * cos(qRoll-boom_mount_angle); 
end

== matlab function spring_mass_model_01/Control/Behavior Control/Torque Distribution Left/Motor Torque Saturation Optimization ==
  data: x1s input; t1 output; x2s input; lambda1 parameter; lambda2 parameter; LEG_MTR_MAX_TORQUE parameter; t2 output
% Optimal leg motor torque distribution
function [t1, t2] = distribute_torque(x1s, x2s, lambda1, lambda2, LEG_MTR_MAX_TORQUE)

s = LEG_MTR_MAX_TORQUE;

% possible solutions
x1 = [                                                      x1s;
                                                            0;
                                                            s;
                                                            0;
                                                           -s;
  (lambda2*s + lambda1*x1s - lambda2*x2s)/(lambda1 + lambda2);
  (lambda1*x1s - lambda2*s + lambda2*x2s)/(lambda1 + lambda2);
  (lambda2*s + lambda1*x1s + lambda2*x2s)/(lambda1 + lambda2);
 -(lambda2*s - lambda1*x1s + lambda2*x2s)/(lambda1 + lambda2)];
 
x2 = [                                                      x2s;
                                                            s;
                                                            0;
                                                           -s;
                                                            0;
  (lambda1*s - lambda1*x1s + lambda2*x2s)/(lambda1 + lambda2);
  (lambda1*s + lambda1*x1s + lambda2*x2s)/(lambda1 + lambda2);
  (lambda1*x1s - lambda1*s + lambda2*x2s)/(lambda1 + lambda2);
 -(lambda1*s + lambda1*x1s - lambda2*x2s)/(lambda1 + lambda2)];

% test constraints
c1 = s - x1 - x2 >= 0;
c2 = s + x1 + x2 >= 0;
c3 = s - x1 + x2 >= 0;
c4 = s + x1 - x2 >= 0;
constraints = c1 & c2 & c3 & c4;

% objective function to maximize
f = -lambda1*(x1-x1s).^2-lambda2*(x2-x2s).^2;
satisfied = find(constraints);
[~,I] = max(f(satisfied));

t1 = x1(satisfied(I));
t2 = x2(satisfied(I));

== matlab function spring_mass_model_01/Control/Behavior Control/Velocity Estimation/Takeoff Velocity/vertical_velocity ==
  data: y output; dx output; dy output double; l input; dl input; phi input; dphi input; qPitch input; dqPitch input; d_y_com parameter
function [y,dx,dy] = fcn(l, dl, phi, dphi, qPitch, dqPitch, d_y_com)

% y = -l*cos(theta+phi) + d*cos(theta)
% dy = -dl*cos(theta+phi) + l*(dtheta+dphi)*sin(theta+phi) - d*dtheta*sin(theta)
gamma = phi + qPitch;
dgamma = dphi + dqPitch;
d = d_y_com;

y = -l*cos(gamma) + d*cos(qPitch);
dy = -dl*cos(gamma) + l*dgamma*sin(gamma) - d*dqPitch*sin(qPitch);

% x = -l*sin(gamma) + d*sin(theta)
% dx = -dl*sin(gamma) - l*dgamma*cos(gamma) + d*dtheta*cos(theta)

dx = -dl*sin(gamma) - l*dgamma*cos(gamma) + d*dqPitch*cos(qPitch);
